simulink model "SMC2"  (R2020a)
settings: Solver=VariableStepAuto  StartTime=0.0  StopTime=10.0  RelTol=1e-3
model workspace (MAT data in the model file):
  A = Simulink.Parameter
  A.Value = Simulink.data.Expression
  A.Value.ExpressionString = "dsys.A"
  A.DataType = 'auto'
  A.Dimensions = -1
  B = Simulink.Parameter
  B.Value = Simulink.data.Expression
  B.Value.ExpressionString = "dsys.B"
  B.DataType = 'auto'
  B.Dimensions = -1
  C = Simulink.Parameter
  C.Value = Simulink.data.Expression
  C.Value.ExpressionString = "[c 1]'"
  C.DataType = 'auto'
  C.Dimensions = -1
  SMC_sdosession_filter : sldodialogs.data.SessionData (value not decoded)
  SMC_sdosession_nofilter : sldodialogs.data.SessionData (value not decoded)
  Ts = 0.02
  c = 0.113153713092
  delta = 0.00542659386424
  g = 0.0160126687884
  k_lp = 0.24
  m = 0.0180335208934
  q = 0.838558181882
  tau_lp = 0.015
undefined symbols (not defined in the file or in its folder): DiscIntNeverNeededParam, m11, x607325_PPR
libraries: simulink_extras x2, eeGeneralControl x1, simulink x1
settings Model: Creator=khoi  LastModifiedBy=khoi

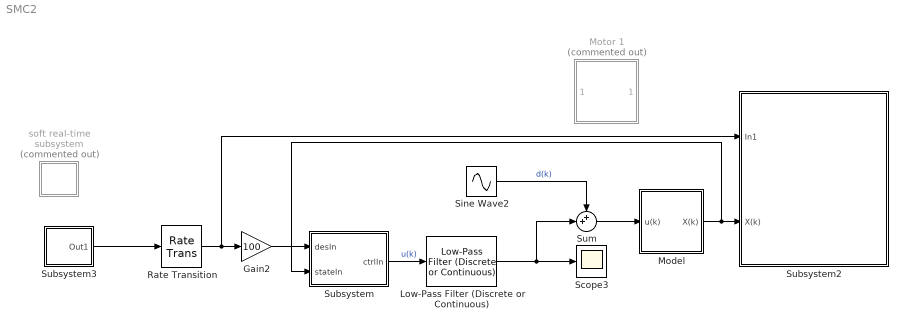
== system SMC2 ==
  Gain2 : Gain  Gain=100
  Low-Pass Filter (Discrete or Continuous) : eeGeneralControl/Low-Pass Filter (Discrete or Continuous)  K=k_lp  T=tau_lp  B=inf  A=-inf  init_option=Inherited from block input  x0=0  Ts=Ts
  Model : Subsystem
  Motor 1 : Subsystem  Commented=on
  Rate Transition : RateTransition  OutPortSampleTime=Ts
  Scope3 : Scope
  Sine Wave2 : Sin  Amplitude=1.5  Frequency=2*pi  SampleTime=Ts
  Subsystem : Subsystem
  Subsystem2 : Subsystem
  Subsystem3 : Subsystem
  Sum : Sum  Inputs=++|
  soft real-time subsystem : Subsystem  Commented=on  mask{t_sample=0.01}
      mask prompts: t_sample "Sleep function interval (s)"
  wires:
  Subsystem3/1(Out1) -> Rate Transition/1
  Sine Wave2/1 -> Sum/1  "d(k)"
  Subsystem/1(ctrlIn) -> Low-Pass Filter (Discrete or Continuous)/1  "u(k)"
  Gain2/1 -> Subsystem/1(desIn)
  Sum/1 -> Model/1(u(k))
  Rate Transition/1 -> Gain2/1, Subsystem2/1(In1)
  Low-Pass Filter (Discrete or Continuous)/1 -> Scope3/1, Sum/2
  Model/1(X(k)) -> Subsystem/2(stateIn), Subsystem2/2(X(k))

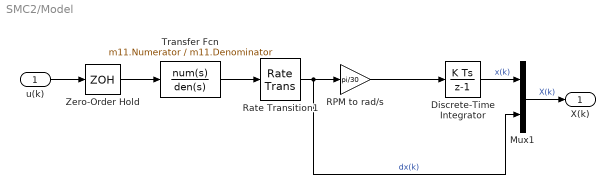
== system SMC2/Model ==
  u(k) : Inport
  Discrete-Time Integrator : DiscreteIntegrator  SampleTime=-1  ICPrevOutput=DiscIntNeverNeededParam  ICPrevScaledInput=DiscIntNeverNeededParam
  Mux1 : Mux  Inputs=2
  RPM to rad/s : Gain  Gain=pi/30
  Rate Transition1 : RateTransition  OutPortSampleTime=Ts
  Transfer Fcn : TransferFcn  Numerator=m11.Numerator  Denominator=m11.Denominator
  Zero-Order Hold : ZeroOrderHold  SampleTime=-1
  X(k) : Outport
  wires:
  Rate Transition1/1 -> Mux1/2, RPM to rad/s/1  "dx(k)"
  u(k)/1 -> Zero-Order Hold/1
  Zero-Order Hold/1 -> Transfer Fcn/1
  RPM to rad/s/1 -> Discrete-Time Integrator/1
  Discrete-Time Integrator/1 -> Mux1/1  "x(k)"
  Transfer Fcn/1 -> Rate Transition1/1
  Mux1/1 -> X(k)/1  "X(k)"

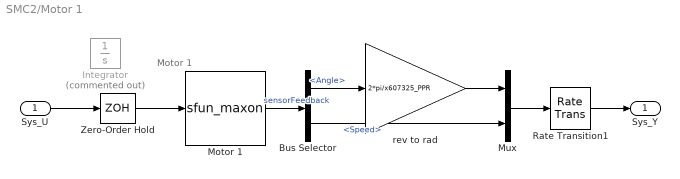
== system SMC2/Motor 1 ==
  note: Motor 1
  Sys_U : Inport
  Bus Selector : BusSelector  OutputSignals=Angle,Speed
  Integrator : Integrator  Commented=on
  Motor 1 : S-Function  FunctionName=sfun_maxon  Parameters=NodeID, DeltaT, OpMode  SFunctionDeploymentMode=off  EnableBusSupport=off  mask{NodeID=1, DeltaT=0.02, OpMode=Cyclic synchronous velocity mode, P_cur=0, I_cur=0, P_pos=0, I_pos=0, D_pos=0, v_posGainFF=0, a_posGainFF=0, P_vel=0, I_vel=0, v_velGainFF=0, a_velGainFF=0, f_velCutoff=0}
      mask prompts: NodeID "Node ID"; DeltaT "Sample time (s)"; OpMode "Operation mode"; P_cur "P gain"; I_cur "I gain"; P_pos "P gain"; I_pos "I gain"; D_pos "D gain"; v_posGainFF "FF velocity gain"; a_posGainFF "FF acceleration gain"; P_vel "P gain"; I_vel "I gain"; v_velGainFF "Feed-forward velocity gain"; a_velGainFF "Feed-forward acceleration gain"; f_velCutoff "Filter cut-off frequency"
      mask TypeOptions OpMode: Cyclic synchronous current (torque) mode | Cyclic synchronous velocity mode | Cyclic synchronous position mode | Profile velocity mode | Profile position mode
      mask DialogControl DescGroupVar Prompt: Motor Parameters
      mask DialogControl DescTextVar Prompt: The block outputs MotorInfo bus signal, which consists of the following variables: angle (increment), speed (rpm), current (mA)
      mask DialogControl Container6 Prompt: Motor
      mask DialogControl Container14 Prompt: Controller Parameters
      mask DialogControl DescTextVar_copy Prompt: This tab is experimental and does not implemented yet. Changing these parameters will not affect the motor performance.
      mask DialogControl Container15 Prompt: Current controller parameter set
      mask DialogControl Container15_copy Prompt: Position controller parameter set
      mask DialogControl Container15_copy_copy Prompt: Velocity controller parameter set
      mask Display:
      | disp('Maxon motor\nHIL');
      | % port_label('input', 1, 'inputSignal');
      | % port_label('output', 1, 'SENSR');
  Mux : Mux  Inputs=2
  Rate Transition1 : RateTransition
  Zero-Order Hold : ZeroOrderHold  SampleTime=-1
  rev to rad : Gain  Gain=2*pi/x607325_PPR
  Sys_Y : Outport
  wires:
  Rate Transition1/1 -> Sys_Y/1
  Zero-Order Hold/1 -> Motor 1/1
  Mux/1 -> Rate Transition1/1
  Bus Selector/2 -> Mux/2  "<Speed>"
  rev to rad/1 -> Mux/1
  Motor 1/1 -> Bus Selector/1  "sensorFeedback"
  Bus Selector/1 -> rev to rad/1  "<Angle>"
  Sys_U/1 -> Zero-Order Hold/1

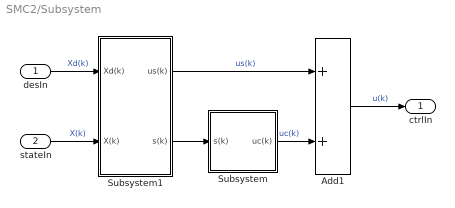
== system SMC2/Subsystem ==
  desIn : Inport
  stateIn : Inport  Port=2
  Add1 : Sum
  Subsystem : Subsystem
  Subsystem1 : Subsystem
  ctrlIn : Outport
  wires:
  Subsystem1/2(s(k)) -> Subsystem/1(s(k))
  Subsystem1/1(us(k)) -> Add1/1  "us(k)"
  stateIn/1 -> Subsystem1/2(X(k))  "X(k)"
  Subsystem/1(uc(k)) -> Add1/2  "uc(k)"
  desIn/1 -> Subsystem1/1(Xd(k))  "Xd(k)"
  Add1/1 -> ctrlIn/1  "u(k)"

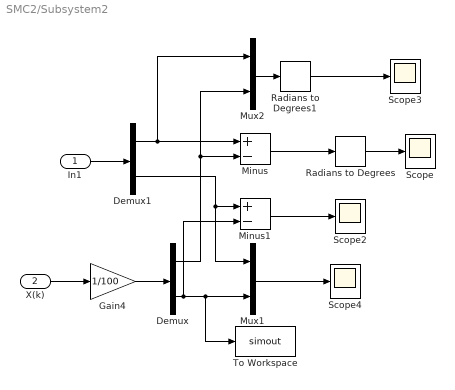
== system SMC2/Subsystem2 ==
  In1 : Inport
  X(k) : Inport  Port=2
  Demux : Demux  Outputs=2
  Demux1 : Demux  Outputs=2
  Gain4 : Gain  Gain=1/100
  Minus : Sum  Inputs=+-
  Minus1 : Sum  Inputs=+-
  Mux1 : Mux  Inputs=2
  Mux2 : Mux  Inputs=2
  Radians to Degrees : simulink_extras/Transformations/Radians to Degrees
  Radians to Degrees1 : simulink_extras/Transformations/Radians to Degrees
  Scope{,2..4} (4 alike) : Scope
  To Workspace : ToWorkspace  VariableName=simout  SaveFormat=Timeseries  SampleTime=-1
  wires:
  Mux1/1 -> Scope4/1
  Radians to Degrees1/1 -> Scope3/1
  Demux/1 -> Mux2/2, Minus/2
  Minus1/1 -> Scope2/1
  Minus/1 -> Radians to Degrees/1
  Gain4/1 -> Demux/1
  Radians to Degrees/1 -> Scope/1
  Demux1/1 -> Mux2/1, Minus/1
  Mux2/1 -> Radians to Degrees1/1
  Demux1/2 -> Mux1/1, Minus1/1
  X(k)/1 -> Gain4/1
  Demux/2 -> To Workspace/1, Mux1/2, Minus1/2
  In1/1 -> Demux1/1

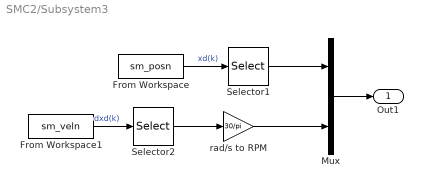
== system SMC2/Subsystem3 ==
  From Workspace : FromWorkspace  VariableName=sm_posn
  From Workspace1 : FromWorkspace  VariableName=sm_veln
  Mux : Mux  Inputs=2
  Selector1 : Selector  InputPortWidth=4  IndexOptions=Index vector (dialog)  Indices=1  OutputSizes=1
  Selector2 : Selector  InputPortWidth=4  IndexOptions=Index vector (dialog)  Indices=1  OutputSizes=1
  rad/s to RPM : Gain  Gain=30/pi
  Out1 : Outport
  wires:
  From Workspace1/1 -> Selector2/1  "dxd(k)"
  Selector1/1 -> Mux/1
  rad/s to RPM/1 -> Mux/2
  From Workspace/1 -> Selector1/1  "xd(k)"
  Mux/1 -> Out1/1
  Selector2/1 -> rad/s to RPM/1

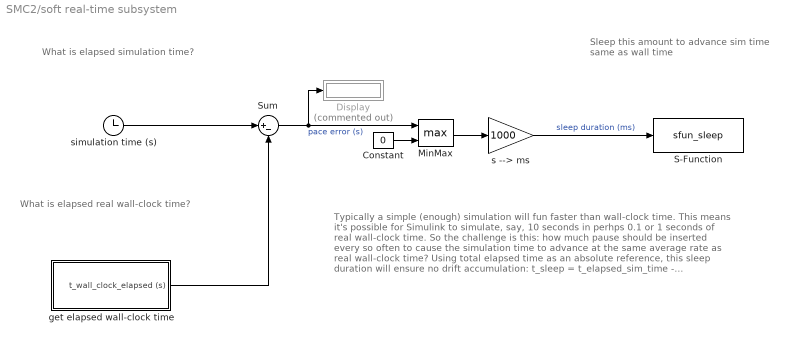
== system SMC2/soft real-time subsystem ==
  note: What is elapsed real
      | wall-clock time?
  note: What is elapsed
      | simulation time?
  note: Sleep this amount
      | to advance sim time
      | same as wall time
  note: Typically a simple (enough) simulation will fun faster than
      | wall-clock time. This means it's possible for Simulink to
      | simulate, say, 10 seconds in perhps 0.1 or 1 seconds of real
      | wall-clock time.
      |
      | So the challenge is this: how much pause should be inserted
      | every so often to cause the simulation time to advance at
      | the same average rate as real wall-clock time?
      |
      | Using total elapsed time as an absolute reference, this
      | sleep duration will ensure no drift accumulation:
      |
      | t_sleep = t_elapsed_sim_time - t_elapsed_wall_clock_time
      |
      | Pace error and Sleep() or usleep() resolution is system dependent
      | and likely around 10ms on Windows machines. Better on linux.
      |
      | Marc Compere
      | comperem@gmail.com
      | created : 28 May 2018
      | modified: 29 May 2018
      |
      | Reference:
      | Marc Compere (2022). S oft Real Time Block for Pacing Simulink Simulations (https://www.mathworks.com/matlabcentral/fileexchange/67520-soft-real-time-block-for-pacing-simulink-simulations), MATLAB Central File Exchange. Retrieved March 14, 2022.
  Constant : Constant  Value=0
  Display : Display  Commented=on
  MinMax : MinMax  Function=max  Inputs=2
  S-Function : S-Function  FunctionName=sfun_sleep  Parameters=t_sample  SFunctionDeploymentMode=off  EnableBusSupport=off
  Sum : Sum  Inputs=|+-
  get elapsed wall-clock time : Subsystem
  s --> ms : Gain  Gain=1000
  simulation time (s) : Clock
  wires:
  simulation time (s)/1 -> Sum/1
  Constant/1 -> MinMax/2
  get elapsed wall-clock time/1(t_wall_clock_elapsed (s)) -> Sum/2
  Sum/1 -> Display/1, MinMax/1  "pace error (s)"
  MinMax/1 -> s --> ms/1
  s --> ms/1 -> S-Function/1  "sleep duration (ms)"

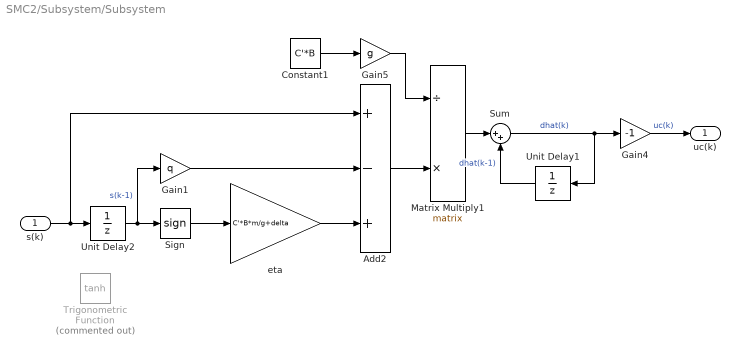
== system SMC2/Subsystem/Subsystem ==
  s(k) : Inport
  Add2 : Sum  Inputs=+-+
  Constant1 : Constant  Value=C'*B
  Gain1 : Gain  Gain=q
  Gain4 : Gain  Gain=-1
  Gain5 : Gain  Gain=g
  Matrix Multiply1 : Product  Inputs=/*  Multiplication=Matrix(*)
  Sign : Signum
  Sum : Sum  Inputs=|++
  Trigonometric Function : Trigonometry  Commented=on  Operator=tanh
  Unit Delay1 : UnitDelay  SampleTime=-1  HasFrameUpgradeWarning=on
  Unit Delay2 : UnitDelay  SampleTime=-1  HasFrameUpgradeWarning=on
  eta : Gain  Gain=C'*B*m/g+delta
  uc(k) : Outport
  wires:
  Add2/1 -> Matrix Multiply1/2
  Constant1/1 -> Gain5/1
  Gain1/1 -> Add2/2
  Gain4/1 -> uc(k)/1  "uc(k)"
  Gain5/1 -> Matrix Multiply1/1
  Unit Delay1/1 -> Sum/2  "dhat(k-1)"
  Matrix Multiply1/1 -> Sum/1
  Sum/1 -> Unit Delay1/1, Gain4/1  "dhat(k)"
  Sign/1 -> eta/1
  eta/1 -> Add2/3
  s(k)/1 -> Add2/1, Unit Delay2/1
  Unit Delay2/1 -> Sign/1, Gain1/1  "s(k-1)"

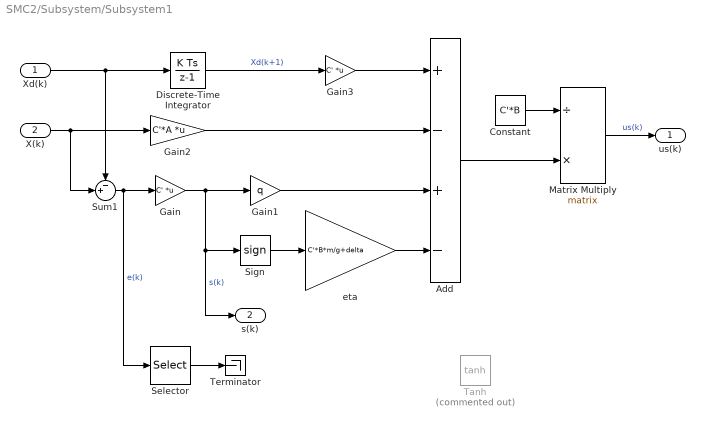
== system SMC2/Subsystem/Subsystem1 ==
  Xd(k) : Inport
  X(k) : Inport  Port=2
  Add : Sum  Inputs=+-+-
  Constant : Constant  Value=C'*B
  Discrete-Time Integrator : DiscreteIntegrator  SampleTime=-1  ICPrevOutput=DiscIntNeverNeededParam  ICPrevScaledInput=DiscIntNeverNeededParam
  Gain : Gain  Gain=C'  Multiplication=Matrix(K*u)
  Gain1 : Gain  Gain=q
  Gain2 : Gain  Gain=C'*A  Multiplication=Matrix(K*u)
  Gain3 : Gain  Gain=C'  Multiplication=Matrix(K*u)
  Matrix Multiply : Product  Inputs=/*  Multiplication=Matrix(*)
  Selector : Selector  InputPortWidth=2  IndexOptions=Index vector (dialog)  Indices=2  OutputSizes=1
  Sign : Signum
  Sum1 : Sum  Inputs=-+|
  Tanh : Trigonometry  Commented=on  Operator=tanh
  Terminator : Terminator
  eta : Gain  Gain=C'*B*m/g+delta
  us(k) : Outport
  s(k) : Outport  Port=2
  wires:
  Sign/1 -> eta/1
  Matrix Multiply/1 -> us(k)/1  "us(k)"
  eta/1 -> Add/4
  Gain2/1 -> Add/2
  Sum1/1 -> Selector/1, Gain/1  "e(k)"
  Constant/1 -> Matrix Multiply/1
  Gain1/1 -> Add/3
  Gain3/1 -> Add/1
  Add/1 -> Matrix Multiply/2
  Xd(k)/1 -> Sum1/1, Discrete-Time Integrator/1
  X(k)/1 -> Gain2/1, Sum1/2
  Gain/1 -> Sign/1, s(k)/1, Gain1/1  "s(k)"
  Discrete-Time Integrator/1 -> Gain3/1  "Xd(k+1)"
  Selector/1 -> Terminator/1

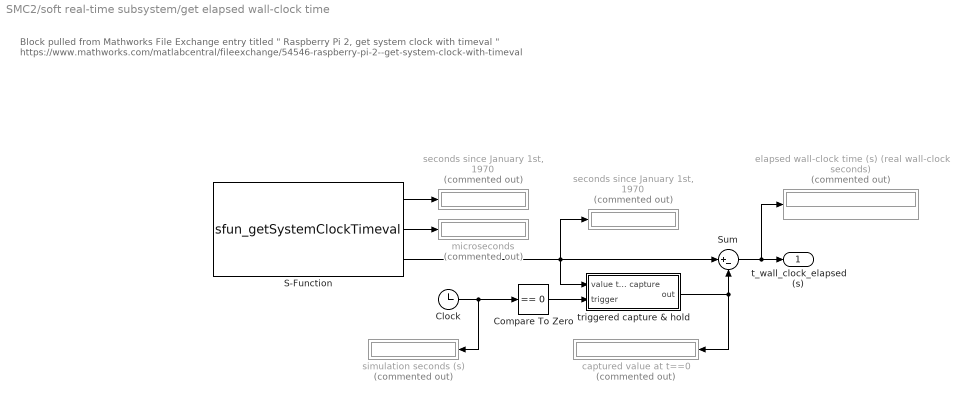
== system SMC2/soft real-time subsystem/get elapsed wall-clock time ==
  note: Block pulled from Mathworks File Exchange entry titled " Raspberry Pi 2, get system clock with timeval "
      |
      | https://www.mathworks.com/matlabcentral/fileexchange/54546-raspberry-pi-2--get-system-clock-with-timeval
  Clock : Clock
  Compare To Zero : simulink/Logic and Bit Operations/Compare To Zero  relop===  OutDataTypeStr=boolean
  S-Function : S-Function  FunctionName=sfun_getSystemClockTimeval  SFunctionDeploymentMode=off  EnableBusSupport=off
  Sum : Sum  Inputs=|+-
  captured value at t==0 : Display  Commented=on
  elapsed wall-clock time (s) (real wall-clock seconds) : Display  Commented=on
  microseconds : Display  Commented=on
  "seconds since January 1st, 1970" : Display  Commented=on
  "seconds since January 1st, 1970 " : Display  Commented=on
  simulation seconds (s) : Display  Commented=on
  triggered capture & hold : Subsystem
  t_wall_clock_elapsed (s) : Outport
  wires:
  triggered capture & hold/1(out) -> captured value at t==0/1, Sum/2
  S-Function/1 -> "seconds since January 1st, 1970 "/1
  Compare To Zero/1 -> triggered capture & hold/2(trigger)
  Sum/1 -> t_wall_clock_elapsed (s)/1, elapsed wall-clock time (s) (real wall-clock seconds)/1
  S-Function/2 -> microseconds/1
  S-Function/3 -> triggered capture & hold/1(value to capture), Sum/1, "seconds since January 1st, 1970"/1
  Clock/1 -> Compare To Zero/1, simulation seconds (s)/1

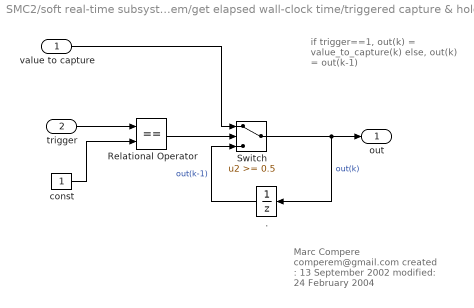
== system SMC2/soft real-time subsystem/get elapsed wall-clock time/triggered capture & hold ==
  note: Marc Compere
      | comperem@gmail.com
      | created  : 13 September 2002
      | modified: 24 February 2004
  note: if trigger==1,
      |    out(k) = value_to_capture(k)
      | else,
      |    out(k) = out(k-1)
  value to capture : Inport
  trigger : Inport  Port=2
  . : UnitDelay  SampleTime=-1  HasFrameUpgradeWarning=on
  Relational Operator : RelationalOperator  Operator===  RndMeth=Nearest
  Switch : Switch  Threshold=0.5  SaturateOnIntegerOverflow=on
  const : Constant
  out : Outport
  wires:
  trigger/1 -> Relational Operator/1
  const/1 -> Relational Operator/2
  Relational Operator/1 -> Switch/2
  Switch/1 -> ./1, out/1  "out(k)"
  value to capture/1 -> Switch/1
  ./1 -> Switch/3  "out(k-1)"
